simulink model "Anillos_SimExam2"  (R2021a)
settings: Solver=ode45  StartTime=0.0  StopTime=20.0  RelTol=1e-3  EnableMultiTasking=on
values from neighbouring files (symbols this model uses):
  A = [0 -pS(3) ... (first row only)    [ej4.m]
  B = [1 -pSR(2) ... (first row only)    [ej4.m]
  C = [0 1]    [ej4.m]
  D = [0 -pR(1)]    [ej4.m]
  gg = double(subs(FT,s,0))    [ej4.m]
  M = collect(s^3-s,s)    [MatlabDivisionEuclides.m]    (also in ej4.m = sym2poly(collect(s^3-s,s)))
  N = -4*s^2+1    [MatlabDivisionEuclides.m]    (also in ej4.m = [0 -4     0     1])
settings Model: Creator=Tlayekanketl  LastModifiedBy=Idael
settings SolverCC: AlgebraicLoopSolver=TrustRegion
settings DataIOCC: LimitDataPoints=on  SaveFormat=Array  ReturnWorkspaceOutputs=off
settings OptimizationCC: LifeSpan=inf
settings DebuggingCC: UnderspecifiedInitializationDetection=Classic  MergeDetectMultiDrivingBlocksExec=none  AllowSymbolicDim=off  StateNameClashWarn=warning  SFUnexpectedBacktrackingDiag=warning  SFNoUnconditionalDefaultTransitionDiag=warning  SFExecutionAtInitializationDiag=none  SFMachineParentedDataDiag=warning  ArithmeticOperatorsInVariantConditions=warning
settings HardwareCC: ProdBitPerPointer=32  ProdBitPerSizeT=32  ProdBitPerPtrDiffT=32  ProdLargestAtomicFloat=None  ProdIntDivRoundTo=Undefined  ProdEndianess=Unspecified  ProdWordSize=32  ProdHWDeviceType=32-bit Generic
settings ModelReferenceCC: PropagateSignalLabelsOutOfModel=off
settings SFSimCC: SimUseLocalCustomCode=off  CustomCodeUndefinedFunction=UseInterfaceOnly
settings RTWCC: RTWUseLocalCustomCode=off
settings CodeAppCC: StateflowObjectComments=on
settings GRTTargetCC: TargetLangStandard=C89/C90 (ANSI)
settings ConfigComp: CovMetricSettings=dw  CovSaveCumulativeToWorkspaceVar=on  CovSaveSingleToWorkspaceVar=on  CovExternalEMLEnable=off  CovSFcnEnable=off

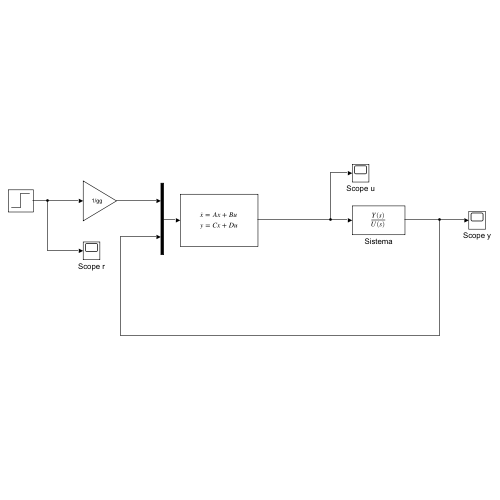
[thumbnail: Simulink's stored preview of the top-level diagram]
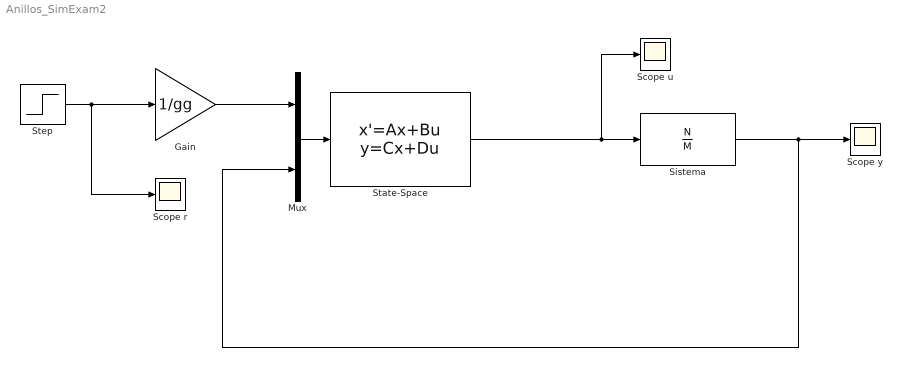
== system Anillos_SimExam2 ==
  Gain : Gain  Gain=1/gg
  Mux : Mux  Inputs=2
  Scope r : Scope
  Scope u : Scope
  Scope y : Scope
  Sistema : TransferFcn  Numerator=N  Denominator=M
  State-Space : StateSpace  A=A  B=B  C=C  D=D  InitialCondition=0
  Step : Step  SampleTime=0
  wires:
  Step/1 -> Gain/1, Scope r/1
  Sistema/1 -> Scope y/1, Mux/2
  State-Space/1 -> Scope u/1, Sistema/1
  Gain/1 -> Mux/1
  Mux/1 -> State-Space/1
